simulink model "pendulo_duplo"  (R2015b)
settings: Solver=VariableStepAuto  StartTime=0.0  RelTol=1e-3
values from neighbouring files (symbols this model uses):
  g = 9.8    [Lab1.m]
  l = 0.5    [Lab1.m]
  m = 1    [Lab1.m]
  p_1_inicial = (1/6)*m*(l^2)*(3*dteta2*cos(teta_1_inicial-teta_2_inicial))    [Lab1.m]
  p_2_inicial = (1/6)*m*(l^2)*(2*dteta2)    (= -0.0436332312999)    [Lab1.m]
  teta_1_inicial = teta(1)    [Lab1.m]
  teta_2_inicial = teta(2)    [Lab1.m]
settings Model: Creator=Alice  LastModifiedBy=Alice

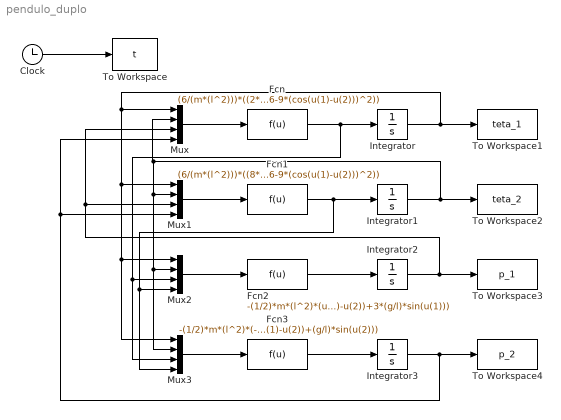
== system pendulo_duplo ==
  Clock : Clock
  Fcn : Fcn  Expr=(6/(m*(l^2)))*((2*u(3)-3*cos(u(1)-u(2))*u(4))/(16-9*(cos(u(1)-u(2)))^2))
  Fcn1 : Fcn  Expr=(6/(m*(l^2)))*((8*u(4)-3*cos(u(1)-u(2))*u(3))/(16-9*(cos(u(1)-u(2)))^2))
  Fcn2 : Fcn  Expr=-(1/2)*m*(l^2)*(u(3)*u(4)*sin(u(1)-u(2))+3*(g/l)*sin(u(1)))
  Fcn3 : Fcn  Expr=-(1/2)*m*(l^2)*(-u(3)*u(4)*sin(u(1)-u(2))+(g/l)*sin(u(2)))
  Integrator : Integrator  InitialCondition=teta_1_inicial
  Integrator1 : Integrator  InitialCondition=teta_2_inicial
  Integrator2 : Integrator  InitialCondition=p_1_inicial
  Integrator3 : Integrator  InitialCondition=p_2_inicial
  Mux{,1..3} (4 alike) : Mux
  To Workspace : ToWorkspace  VariableName=t  SampleTime=0.001
      settings: Decimation=10
  To Workspace1 : ToWorkspace  VariableName=teta_1  SampleTime=0.001
      settings: Decimation=10
  To Workspace2 : ToWorkspace  VariableName=teta_2  SampleTime=0.001
      settings: Decimation=10
  To Workspace3 : ToWorkspace  VariableName=p_1  SampleTime=0.001
      settings: Decimation=10
  To Workspace4 : ToWorkspace  VariableName=p_2  SampleTime=0.001
      settings: Decimation=10
  wires:
  Clock/1 -> To Workspace/1
  Mux/1 -> Fcn/1
  Mux1/1 -> Fcn1/1
  Mux2/1 -> Fcn2/1
  Mux3/1 -> Fcn3/1
  Fcn/1 -> Mux3/3, Mux2/3, Integrator/1
  Fcn1/1 -> Mux2/4, Mux3/4, Integrator1/1
  Fcn2/1 -> Integrator2/1
  Fcn3/1 -> Integrator3/1
  Integrator3/1 -> Mux1/4, Mux/4, To Workspace4/1
  Integrator2/1 -> Mux1/3, Mux/3, To Workspace3/1
  Integrator1/1 -> Mux3/2, Mux2/2, Mux1/2, Mux/2, To Workspace2/1
  Integrator/1 -> Mux/1, Mux3/1, Mux2/1, Mux1/1, To Workspace1/1
